simulink model "pitch_loop"  (R2014b)
settings: Solver=ode45  StartTime=0.0  StopTime=10.0  MaxStep=0.1  RelTol=1e-3
undefined symbols (not defined in the file or in its folder): a_theta_1, a_theta_2, a_theta_3, k_d_theta, k_p_theta
settings Model: Creator=kunalmenda  LastModifiedBy=kunalmenda

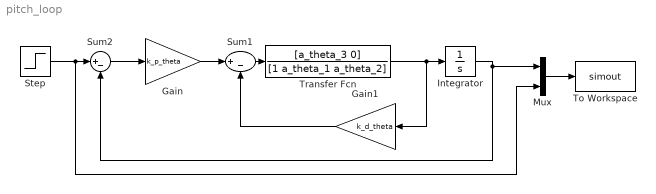
== system pitch_loop ==
  Gain : Gain  Gain=k_p_theta
  Gain1 : Gain  Gain=k_d_theta
  Integrator : Integrator
  Mux : Mux  Inputs=2
  Step : Step  After=10*pi/180  SampleTime=0
  Sum1 : Sum  Inputs=|+-
  Sum2 : Sum  Inputs=|+-
  To Workspace : ToWorkspace  VariableName=simout  SaveFormat=Timeseries  SampleTime=-1
  Transfer Fcn : TransferFcn  Numerator=[a_theta_3 0]  Denominator=[1 a_theta_1 a_theta_2]
  wires:
  Sum2/1 -> Gain/1
  Transfer Fcn/1 -> Gain1/1, Integrator/1
  Sum1/1 -> Transfer Fcn/1
  Integrator/1 -> Mux/1, Sum2/2
  Step/1 -> Mux/2, Sum2/1
  Gain1/1 -> Sum1/2
  Mux/1 -> To Workspace/1
  Gain/1 -> Sum1/1
